simulink model "pfd_connector_example"  (R2022a)
settings: Solver=ode4  StartTime=0.0  StopTime=60  FixedStep=0.03  RelTol=1e-3
libraries: simulink_extras x3
settings Model: Creator=kboychev  LastModifiedBy=kboychev
settings SolverCC: AlgebraicLoopSolver=TrustRegion
settings DataIOCC: ReturnWorkspaceOutputs=off
settings DebuggingCC: UnconnectedInputMsg=warning  UnconnectedOutputMsg=warning  UnconnectedLineMsg=warning  SFMachineParentedDataDiag=warning  ArithmeticOperatorsInVariantConditions=warning
settings SFSimCC: CustomCodeUndefinedFunction=UseInterfaceOnly

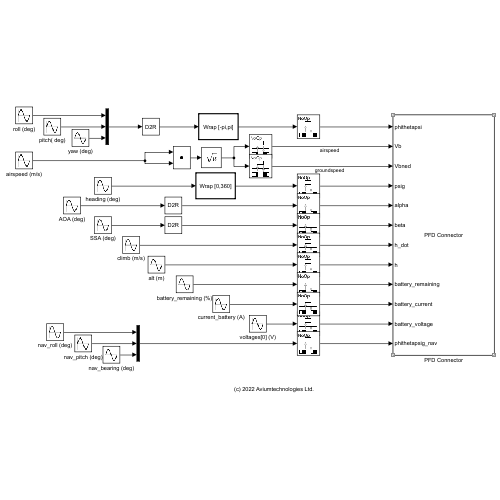
[thumbnail: Simulink's stored preview of the top-level diagram]
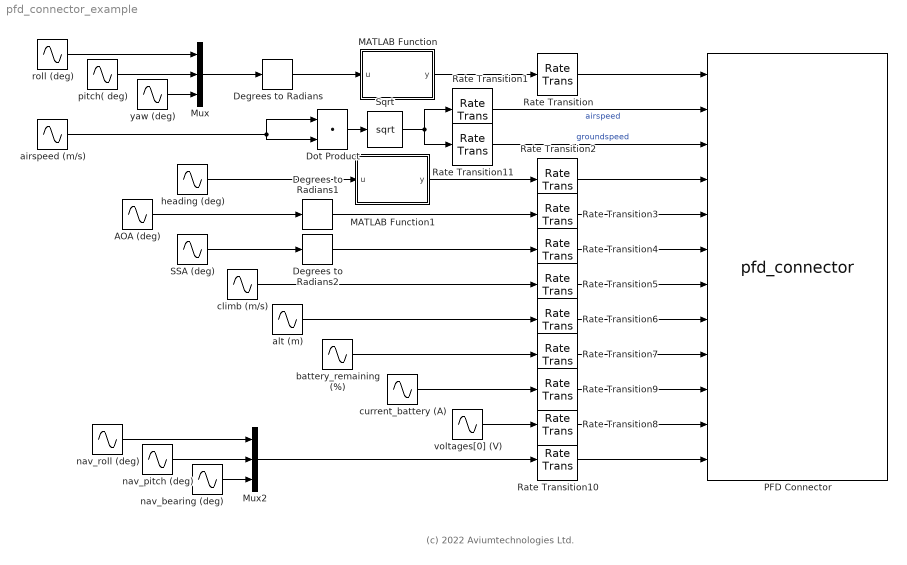
== system pfd_connector_example ==
  note: (c) 2022 Aviumtechnologies Ltd.
  AOA (deg) : Sin  Amplitude=5  SampleTime=0
  Degrees to Radians : simulink_extras/Transformations/Degrees to Radians
  Degrees to Radians1 : simulink_extras/Transformations/Degrees to Radians
  Degrees to Radians2 : simulink_extras/Transformations/Degrees to Radians
  Dot Product : DotProduct  OutDataTypeStr=Inherit: Inherit via internal rule
  MATLAB Function : MATLAB Function  TreatAsAtomicUnit=on
  MATLAB Function1 : MATLAB Function  TreatAsAtomicUnit=on
  Mux : Mux  Inputs=3
  Mux2 : Mux  Inputs=3
  PFD Connector : S-Function  FunctionName=pfd_connector  SFunctionDeploymentMode=off  EnableBusSupport=off  mask(HUD Connector){}
      mask help: A block that sends the aircraft's position, orientation, airspeed and groundspeed in a JSON format to a heads-up-display (HUD) application for visualization. Uses the Asio C++ library for UDP sockets. You can download the HUD application from here:
      mask Display:
      | fprintf('PFD Connector');
      | port_label('input',1,'phithetapsi');
      | port_label('input',2,'Vb');
      | port_label('input',3,'Vbned');
      | port_label('input',4,'psig');
      | port_label('input',5,'alpha');
      | port_label('input',6,'beta');
      | port_label('input',7,'h_dot');
      | port_label('input',8,'h');
      | port_label('input',9,'battery_remaining');
      | port_label('input',10,'battery_current');
      | port_label('input',11,'battery_voltage');
      | port_label('input',12,'phithetapsig_nav');
  Rate Transition{,1..11} (12 alike) : RateTransition  OutPortSampleTime=0.03
  SSA (deg) : Sin  Amplitude=3  SampleTime=0
  Sqrt : Sqrt
  airspeed (m/s) : Sin  Amplitude=[2 0 0]  Bias=[25 0 0]  SampleTime=0
  alt (m) : Sin  Amplitude=10  Bias=1000  SampleTime=0
  battery_remaining (%) : Sin  Amplitude=20  Bias=80  SampleTime=0
  climb (m/s) : Sin  Amplitude=5  SampleTime=0
  current_battery (A) : Sin  Amplitude=5  Bias=30  SampleTime=0
  heading (deg) : Sin  Amplitude=175  Bias=-135  Frequency=0.5  SampleTime=0
  nav_bearing (deg) : Sin  Bias=-135  SampleTime=0
  nav_pitch (deg) : Sin  Bias=5  SampleTime=0
  nav_roll (deg) : Sin  Bias=30  SampleTime=0
  pitch( deg) : Sin  Amplitude=10  SampleTime=0
  roll (deg) : Sin  Amplitude=10  SampleTime=0
  voltages[0] (V) : Sin  Amplitude=0.2  Bias=22.2  SampleTime=0
  yaw (deg) : Sin  Amplitude=180  Bias=-135  Frequency=0.5  SampleTime=0
  wires:
  Mux/1 -> Degrees to Radians/1
  AOA (deg)/1 -> Degrees to Radians1/1
  SSA (deg)/1 -> Degrees to Radians2/1
  yaw (deg)/1 -> Mux/3
  pitch( deg)/1 -> Mux/2
  roll (deg)/1 -> Mux/1
  airspeed (m/s)/1 -> Dot Product/1, Dot Product/2
  Degrees to Radians/1 -> MATLAB Function/1(u)
  Degrees to Radians1/1 -> Rate Transition3/1
  Degrees to Radians2/1 -> Rate Transition4/1
  climb (m/s)/1 -> Rate Transition5/1
  alt (m)/1 -> Rate Transition6/1
  battery_remaining (%)/1 -> Rate Transition7/1
  Sqrt/1 -> Rate Transition11/1, Rate Transition1/1
  Rate Transition/1 -> PFD Connector/1
  Rate Transition1/1 -> PFD Connector/2  "airspeed"
  Rate Transition2/1 -> PFD Connector/4
  Rate Transition3/1 -> PFD Connector/5
  Rate Transition4/1 -> PFD Connector/6
  Rate Transition5/1 -> PFD Connector/7
  Rate Transition6/1 -> PFD Connector/8
  Rate Transition7/1 -> PFD Connector/9
  Rate Transition8/1 -> PFD Connector/11
  Rate Transition9/1 -> PFD Connector/10
  current_battery (A)/1 -> Rate Transition9/1
  voltages[0] (V)/1 -> Rate Transition8/1
  Dot Product/1 -> Sqrt/1
  nav_bearing (deg)/1 -> Mux2/3
  nav_roll (deg)/1 -> Mux2/1
  nav_pitch (deg)/1 -> Mux2/2
  Mux2/1 -> Rate Transition10/1
  Rate Transition10/1 -> PFD Connector/12
  Rate Transition11/1 -> PFD Connector/3  "groundspeed"
  heading (deg)/1 -> MATLAB Function1/1(u)
  MATLAB Function1/1(y) -> Rate Transition2/1
  MATLAB Function/1(y) -> Rate Transition/1

== matlab function pfd_connector_example/MATLAB Function ==
  data: u input; y output
function y = wrap_pi(u)
    
y=zeros(size(u));
for i=1:size(u,1)
 
    min=-pi;
    max=pi;

    if min <= u(i) && u(i) < max
        y(i)=u(i);
    else
        range=max-min;
        wraps=floor((u(i)-min)/range);
        y(i)=u(i)-range*wraps;
    end
end

== matlab function pfd_connector_example/MATLAB Function1 ==
  data: u input; y output
function y = wrap_pi(u)
    
y=zeros(size(u));
for i=1:size(u,1)
 
    min=0;
    max=360;

    if min <= u(i) && u(i) < max
        y(i)=u(i);
    else
        range=max-min;
        wraps=floor((u(i)-min)/range);
        y(i)=u(i)-range*wraps;
    end
end
